simulink model "soc_proc"  (R2023b)
settings: Solver=FixedStepDiscrete  StartTime=0.0  StopTime=10.0  RelTol=1e-3  EnableMultiTasking=on
libraries: prociolib x2
settings Model: Creator=user poco smart  LastModifiedBy=user poco smart
settings SolverCC: ConcurrentTasks=on  AlgebraicLoopSolver=TrustRegion  PositivePriorityOrder=on
settings DataIOCC: SaveFormat=Array  SaveOutput=off  SaveTime=off  ReturnWorkspaceOutputs=off
settings OptimizationCC: PassReuseOutputArgsAs=Individual arguments  MaxStackSize=64  EfficientTunableParamExpr=on
settings DebuggingCC: IntegerOverflowMsg=none  ParameterTunabilityLossMsg=error  UnconnectedInputMsg=warning  UnconnectedOutputMsg=warning  UnconnectedLineMsg=warning  PregeneratedLibrarySubsystemCodeDiagnostic=none  ArithmeticOperatorsInVariantConditions=warning
settings HardwareCC: ProdBitPerPointer=32  ProdBitPerSizeT=32  ProdBitPerPtrDiffT=32  ProdLargestAtomicInteger=Long  ProdLargestAtomicFloat=Double  ProdWordSize=32  ProdLongLongMode=on  ProdHWDeviceType=ARM Compatible->ARM Cortex-A (32-bit)  HardwareBoardFeatureSet=SoCBlockset
settings ModelReferenceCC: EnableRefExpFcnMdlSchedulingChecks=on  ModelReferenceNumInstancesAllowed=Single
settings SFSimCC: SimUseLocalCustomCode=off  MATLABDynamicMemAlloc=off  CustomCodeUndefinedFunction=UseInterfaceOnly
settings RTWCC: Description=Embedded Coder  SystemTargetFile=ert.tlc  HardwareBoard=ZedBoard  TLCOptions="-aInlineSetEventsForThisBaseRateFcn=TLC_FALSE -aSuppressMultiTaskScheduler=TLC_FALSE  -aRateBasedStepFcn=0"  TemplateMakefile=ert_default_tmf  GenerateReport=on  RTWUseLocalCustomCode=off  Toolchain=Linaro AArch32 Linux v6.3.1  BuildConfiguration=Faster Runs  IncludeHyperlinkInReport=on  LaunchReport=on  GenerateTraceInfo=on  GenerateTraceReport=on  GenerateTraceReportSl=on  GenerateTraceReportSf=on  GenerateTraceReportEml=on  DLArmComputeVersion=19.05
settings CodeAppCC: ForceParamTrailComments=on  IgnoreCustomStorageClasses=off  OperatorAnnotations=on  SimulinkDataObjDesc=on  SFDataObjDesc=on  InsertBlockDesc=on
settings ERTTargetCC: ExtModeTransport=2  ExtModeStaticAlloc=on  ExtModeMexFile=ext_xcp  ExtModeIntrfLevel=Level2 - Open
settings ConfigComp: CovBoundaryAbsTol=1.0e-5
settings SettingsController: UseSoCProfilerForTargets=0

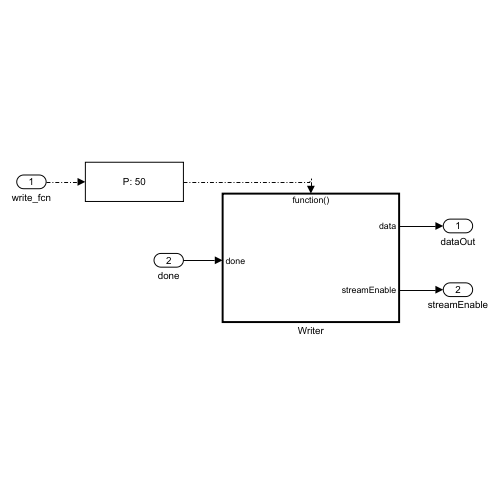
[thumbnail: Simulink's stored preview of the top-level diagram]
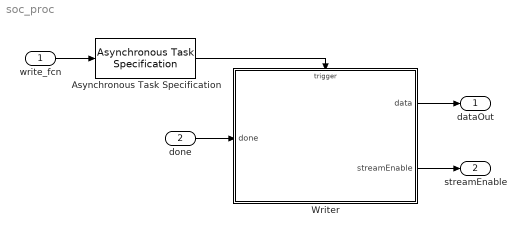
== system soc_proc ==
  write_fcn : Inport  OutputFunctionCall=on
  done : Inport  Port=2  OutDataTypeStr=boolean  PortDimensions=1
  Asynchronous Task Specification : AsynchronousTaskSpecification  TaskPriority=50
  Writer : Subsystem  TreatAsAtomicUnit=on
  dataOut : Outport
  streamEnable : Outport  Port=2
  wires:
  write_fcn/1 -> Asynchronous Task Specification/1
  Asynchronous Task Specification/1 -> Writer/Trigger
  Writer/2(streamEnable) -> streamEnable/1
  done/1 -> Writer/1(done)
  Writer/1(data) -> dataOut/1

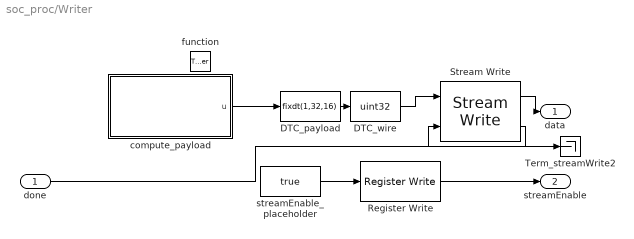
== system soc_proc/Writer ==
  done : Inport  OutDataTypeStr=boolean
  function : TriggerPort  TriggerType=function-call  VariantControl=(inherit)
  DTC_payload : DataTypeConversion  OutDataTypeStr=fixdt(1,32,16)  RndMeth=Floor
  DTC_wire : DataTypeConversion  OutDataTypeStr=uint32  ConvertRealWorld=Stored Integer (SI)  SaturateOnIntegerOverflow=off  RndMeth=Floor
  Register Write : prociolib/Register Write  OutputSink=To output port  TunableParamName=A  RegisterName=streamEnable  DeviceName=/dev/mwipcore  OffsetAddress=hex2dec('0100')  Dummy=0
  Stream Write : prociolib/Stream Write  DeviceName=ip:mm2s  NumberOfBuffers=8  EnableEvent=on
  Term_streamWrite2 : Terminator
  compute_payload : MATLAB Function  TreatAsAtomicUnit=on
  streamEnable_placeholder : Constant  Value=true  OutDataTypeStr=boolean
  data : Outport
  streamEnable : Outport  Port=2
  wires:
  compute_payload/1(u) -> DTC_payload/1
  DTC_payload/1 -> DTC_wire/1
  DTC_wire/1 -> Stream Write/1
  done/1 -> Stream Write/2
  Stream Write/1 -> data/1
  Stream Write/2 -> Term_streamWrite2/1
  streamEnable_placeholder/1 -> Register Write/1
  Register Write/1 -> streamEnable/1

== matlab function soc_proc/Writer/compute_payload ==
  data: u output
function u = compute_payload()
%#codegen
% GENERATO DA build_soc_proc.m â€” non modificare a mano.
% Lato ARM: calcola le due matrici e le impacchetta in 25 elementi.
% Column-major, inverso dell'unpack in soc_fpga (regola R2).

    A = [1 2 3; 4 5 6; 7 8 9];
    B = [9 8 7; 6 5 4; 3 2 1];
    C = [1 2 3 4; 5 6 7 8; 9 10 11 12; 13 14 15 16];
    D = eye(4);

    Y1 = A * B;   % 3x3
    Y2 = C * D;   % 4x4

    u = [reshape(Y1, [], 1); reshape(Y2, [], 1)];   % 9 + 16 = 25
end
